simulink subsystem "Pins"  (R2022a)
settings: Solver=VariableStepAuto  StartTime=0.0  StopTime=10.0  RelTol=1e-3
undefined symbols (not defined in the file or in its folder): D10, D11, D12, D13, D2, D3, D5, D6, D8, D9, PTA0, PTA1, PTA2, PTB9, PTC2, PTC4, PTD0, PTD1, PTD2, PTD3
libraries: frdmk64flib x10
settings Model: Creator=ivanl  LastModifiedBy=ivanl

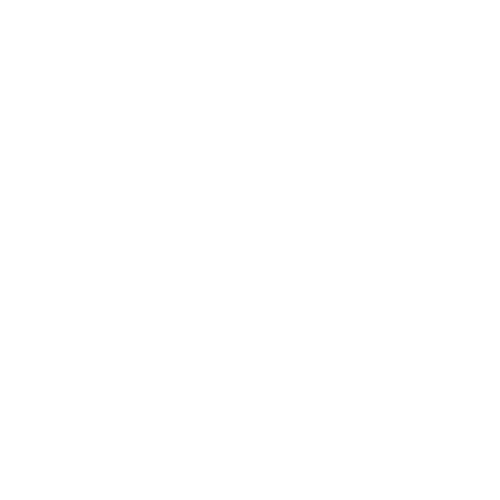
[thumbnail: Simulink's stored preview of the top-level diagram]
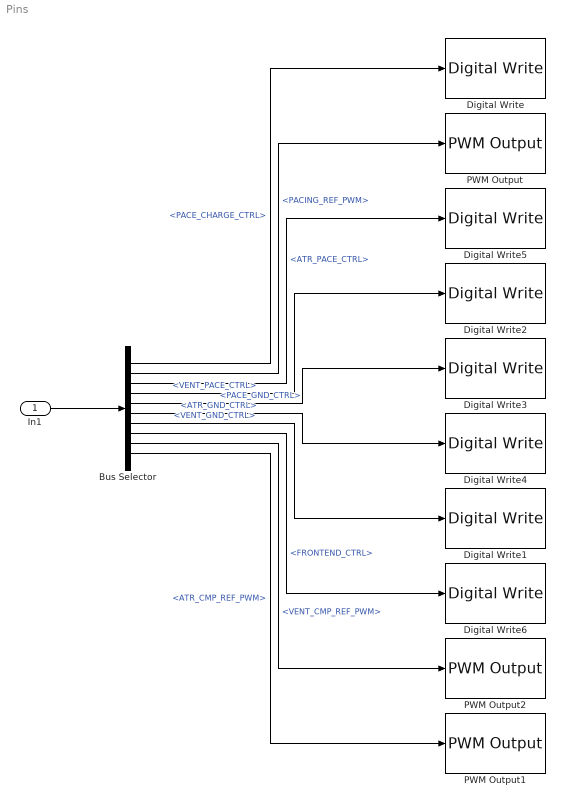
== system Pins ==
  In1 : Inport
  Bus Selector : BusSelector  OutputSignals=PACE_CHARGE_CTRL,PACING_REF_PWM,ATR_PACE_CTRL,VENT_PACE_CTRL,PACE_GND_CTRL,ATR_GND_CTRL,VENT_GND_CTRL,FRONTEND_CTRL,VENT_CMP_REF_PWM,ATR_CMP_REF_PWM
  Digital Write : frdmk64flib/Digital Write  Whichpin=PTB9 (D2)
  Digital Write1 : frdmk64flib/Digital Write  Whichpin=PTD3 (D12)
  Digital Write2 : frdmk64flib/Digital Write  Whichpin=PTC4 (D9)
  Digital Write3 : frdmk64flib/Digital Write  Whichpin=PTD0 (D10)
  Digital Write4 : frdmk64flib/Digital Write  Whichpin=PTD2 (D11)
  Digital Write5 : frdmk64flib/Digital Write  Whichpin=PTA0 (D8)
  Digital Write6 : frdmk64flib/Digital Write  Whichpin=PTD1 (D13)
  PWM Output : frdmk64flib/PWM Output  Whichpin=PTA2 (D5)  InitialFrequency=2000  InitialDutyCycle=0
  PWM Output1 : frdmk64flib/PWM Output  Whichpin=PTC2 (D6)  InitialFrequency=2000  InitialDutyCycle=0
  PWM Output2 : frdmk64flib/PWM Output  Whichpin=PTA1 (D3)  InitialFrequency=2000  InitialDutyCycle=0
  wires:
  In1/1 -> Bus Selector/1
  Bus Selector/1 -> Digital Write/1  "<PACE_CHARGE_CTRL>"
  Bus Selector/2 -> PWM Output/1  "<PACING_REF_PWM>"
  Bus Selector/3 -> Digital Write5/1  "<ATR_PACE_CTRL>"
  Bus Selector/4 -> Digital Write2/1  "<VENT_PACE_CTRL>"
  Bus Selector/5 -> Digital Write3/1  "<PACE_GND_CTRL>"
  Bus Selector/6 -> Digital Write4/1  "<ATR_GND_CTRL>"
  Bus Selector/7 -> Digital Write1/1  "<VENT_GND_CTRL>"
  Bus Selector/8 -> Digital Write6/1  "<FRONTEND_CTRL>"
  Bus Selector/10 -> PWM Output1/1  "<ATR_CMP_REF_PWM>"
  Bus Selector/9 -> PWM Output2/1  "<VENT_CMP_REF_PWM>"
